simulink model "villas_udp"  (Simulink 8.9)
settings: Solver=FixedStepDiscrete  StartTime=0.0  StopTime=inf  FixedStep=0.1  RelTol=1e-3  EnableMultiTasking=on
libraries: simulink x1
settings Model: SuppressorTable=22 serialization::archive 11 0 6 0 0 0 0 0  Creator=stv0g  LastModifiedBy=stv0g
settings DataIOCC: LimitDataPoints=off
settings OptimizationCC: BlockReduction=off  BooleanDataType=off  LifeSpan=auto
settings DebuggingCC: SaveWithParameterizedLinksMsg=none  SignalResolutionControl=TryResolveAllWithWarning  MultiTaskDSMMsg=warning  MultiTaskCondExecSysMsg=none  FcnCallInpInsideContextMsg=error  StateNameClashWarn=none  StrictBusMsg=None  SFUnexpectedBacktrackingDiag=error  SFNoUnconditionalDefaultTransitionDiag=error  SFExecutionAtInitializationDiag=warning
settings HardwareCC: ProdBitPerPointer=64  ProdBitPerSizeT=64  ProdBitPerPtrDiffT=64  ProdLargestAtomicFloat=Float  ProdIntDivRoundTo=Zero  ProdEndianess=LittleEndian  ProdWordSize=64  ProdHWDeviceType=Intel->x86-64 (Windows64)  TargetUnknown=on
settings GRTTargetCC: GeneratePreprocessorConditionals=Use local settings
settings ConfigComp: CovMetricSettings=dwe  CovHtmlReporting=off  CovSaveCumulativeToWorkspaceVar=off  CovSaveSingleToWorkspaceVar=off  CovExternalEMLEnable=on

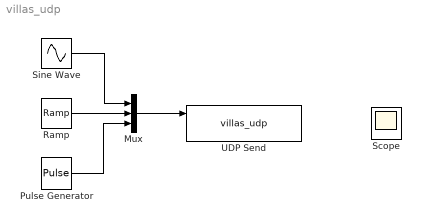
== system villas_udp ==
  Mux : Mux  Inputs=3
  Pulse Generator : DiscretePulseGenerator  PulseType=Time based  Period=10  PulseWidth=5
  Ramp : simulink/Sources/Ramp  slope=1  start=0  X0=0
  Scope : Scope
  Sine Wave : Sin  SampleTime=0
  UDP Send : S-Function  FunctionName=villas_udp  Parameters=local_host,remote_host,local_port,remote_port  SFunctionDeploymentMode=off  EnableBusSupport=off  mask(VILLAS UDP){local_host=127.0.0.1, local_port=64000, remote_host=127.0.0.1, remote_port=64000}
      mask prompts: local_host "Hostname / IP"; local_port "Port"; remote_host "Hostname / IP"; remote_port "Port"
      mask help: This Block exchanges floating point sample data with VILLASnode.
  wires:
  Sine Wave/1 -> Mux/1
  Mux/1 -> UDP Send/1
  Pulse Generator/1 -> Mux/3
  Ramp/1 -> Mux/2
